simulink model "inv_dyn_joint_operational"  (R2023a)
settings: Solver=VariableStepAuto  StartTime=0.0  StopTime=tf  RelTol=1e-3
undefined symbols (not defined in the file): dqi, Kd, Kp, qi, robot
settings Model: Creator=franc  LastModifiedBy=franc

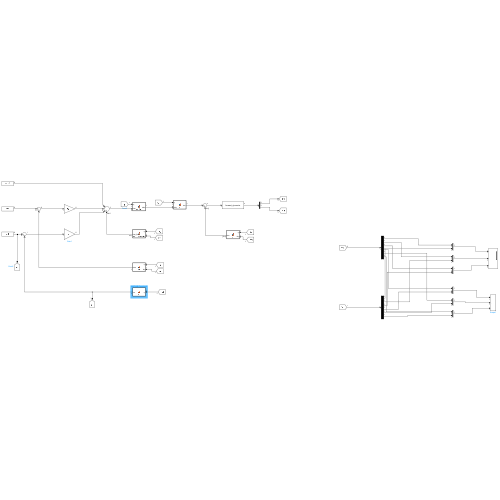
[thumbnail: Simulink's stored preview of the top-level diagram]
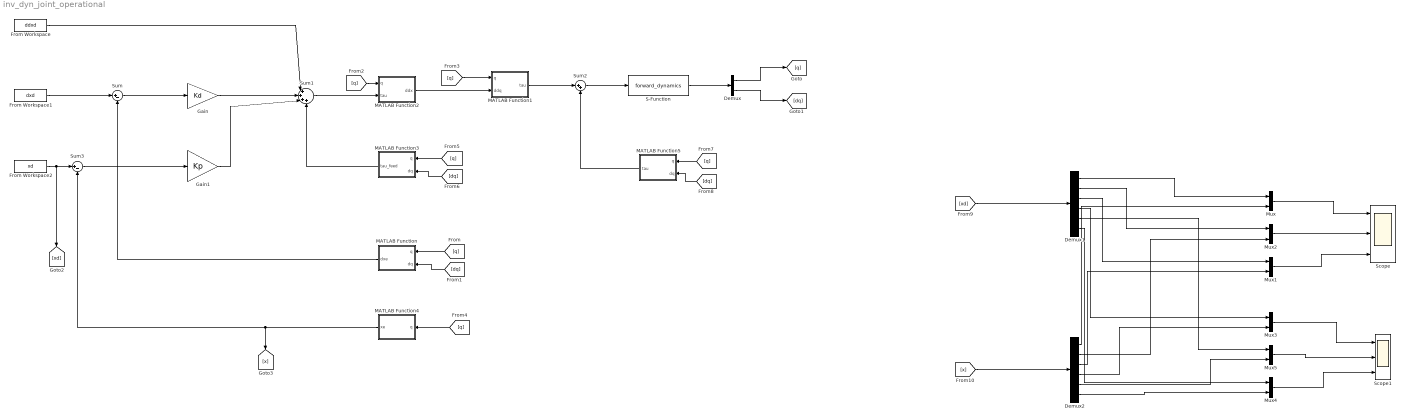
== system inv_dyn_joint_operational ==
  Demux : Demux  Outputs=2
  Demux1 : Demux  Outputs=6
  Demux2 : Demux  Outputs=6
  From Workspace : FromWorkspace  VariableName=ddxd
  From Workspace1 : FromWorkspace  VariableName=dxd
  From Workspace2 : FromWorkspace  VariableName=xd
  Gain : Gain  Gain=Kd
  Gain1 : Gain  Gain=Kp
  MATLAB Function : MATLAB Function  TreatAsAtomicUnit=on
  MATLAB Function1 : MATLAB Function  TreatAsAtomicUnit=on
  MATLAB Function2 : MATLAB Function  TreatAsAtomicUnit=on
  MATLAB Function3 : MATLAB Function  TreatAsAtomicUnit=on
  MATLAB Function4 : MATLAB Function  TreatAsAtomicUnit=on
  MATLAB Function5 : MATLAB Function  TreatAsAtomicUnit=on
  Mux{,1..5} (6 alike) : Mux  Inputs=2
  S-Function : S-Function  FunctionName=forward_dynamics  Parameters=robot,qi,dqi  SFunctionDeploymentMode=off  EnableBusSupport=off
  Scope : Scope  NumInputPorts=3
  Scope1 : Scope  NumInputPorts=3
  Sum : Sum  Inputs=|+-
  Sum1 : Sum  Inputs=|++++
  Sum2 : Sum  Inputs=|++
  Sum3 : Sum  Inputs=|+-
  wires:
  From Workspace1/1 -> Sum/1
  Sum/1 -> Gain/1
  MATLAB Function/1(dxe) -> Sum/2
  [q] -> MATLAB Function/1(q)
  [dq] -> MATLAB Function/2(dq)
  Gain/1 -> Sum1/2
  Gain1/1 -> Sum1/3
  From Workspace/1 -> Sum1/1
  MATLAB Function1/1(tau) -> Sum2/1
  Sum2/1 -> S-Function/1
  Sum1/1 -> MATLAB Function2/2(tau)
  MATLAB Function2/1(ddx) -> MATLAB Function1/2(ddq)
  S-Function/1 -> Demux/1
  Demux/2 -> [dq]
  Demux/1 -> [q]
  [q] -> MATLAB Function2/1(q)
  [q] -> MATLAB Function1/1(q)
  MATLAB Function3/1(tau_feed) -> Sum1/4
  From Workspace2/1 -> Sum3/1, [xd]
  Sum3/1 -> Gain1/1
  MATLAB Function4/1(xe) -> [x], Sum3/2
  [q] -> MATLAB Function4/1(q)
  [q] -> MATLAB Function3/1(q)
  [dq] -> MATLAB Function3/2(dq)
  MATLAB Function5/1(tau) -> Sum2/2
  [q] -> MATLAB Function5/1(q)
  [dq] -> MATLAB Function5/2(dq)
  [xd] -> Demux1/1
  [x] -> Demux2/1
  Demux1/1 -> Mux/1
  Demux1/2 -> Mux2/1
  Demux1/3 -> Mux1/1
  Demux1/4 -> Mux3/1
  Demux1/5 -> Mux5/1
  Demux1/6 -> Mux4/1
  Demux2/1 -> Mux/2
  Demux2/2 -> Mux2/2
  Demux2/3 -> Mux1/2
  Demux2/4 -> Mux3/2
  Demux2/5 -> Mux5/2
  Demux2/6 -> Mux4/2
  Mux3/1 -> Scope1/1
  Mux5/1 -> Scope1/2
  Mux4/1 -> Scope1/3
  Mux/1 -> Scope/1
  Mux2/1 -> Scope/2
  Mux1/1 -> Scope/3

== matlab function inv_dyn_joint_operational/MATLAB Function ==
  data: q input; dxe output; dq input
function dxe = Ja(q,dq)

dxe = zeros(6,1);
dxe = get_Ja_as_9(q(1),q(2),q(3))*dq;

== matlab function inv_dyn_joint_operational/MATLAB Function2 ==
  data: q input; ddx output; tau input
function ddx = Ja_inv(q,tau)

ddx = zeros(3,1);
ddx = get_Ja_inverse_as_9(q(1),q(2),q(3))*tau;

== matlab function inv_dyn_joint_operational/MATLAB Function3 ==
  data: q input; tau_feed output; dq input
function tau_feed = Ja_derivative(q,dq)

tau_feed = zeros(6,1);
tau_feed = get_derivative_Ja_as_9(q(1),q(2),q(3),dq(1),dq(2),dq(3))*dq;

== matlab function inv_dyn_joint_operational/MATLAB Function4 ==
  data: q input; xe output
function xe = K(q)

xe = zeros(6,1);
xe = get_k_as_9(q(1),q(2),q(3));

== matlab function inv_dyn_joint_operational/MATLAB Function5 ==
  data: q input; tau output; dq input
function tau = n(q,dq)
tau = zeros(3,1);
tau = get_n_as_7(q(1),q(3),dq(1),dq(3));

== matlab function inv_dyn_joint_operational/MATLAB Function1 ==
  data: q input; tau output; ddq input
function tau = B(q,ddq)

tau = zeros(3,1);
tau = get_B_as_7(q(1),q(3)) * ddq;
